simulink model "halfcarmodel"  (R2020b)
settings: Solver=VariableStepAuto  StartTime=0.0  StopTime=10.0  RelTol=1e-3
values from neighbouring files (symbols this model uses):
  a = 1.5    [halfcarparameters.mat]
  b = 1    [accel_jerk_ctrl_testbed.m]    (also in halfcarparameters.mat = 1.5)
  K_tf = 201021    [halfcarparameters.mat]
  K_tr = 201021    [halfcarparameters.mat]
  m_s = 879.35    [halfcarparameters.mat]
settings Model: Creator=anishabhangui  LastModifiedBy=anishabhangui

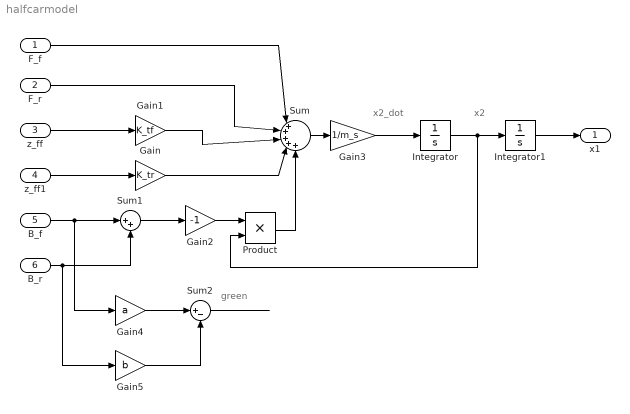
== system halfcarmodel ==
  note: green
  note: x2
  note: x2_dot
  F_f : Inport
  F_r : Inport  Port=2
  z_ff : Inport  Port=3
  z_ff1 : Inport  Port=4
  B_f : Inport  Port=5
  B_r : Inport  Port=6
  Gain : Gain  Gain=K_tr
  Gain1 : Gain  Gain=K_tf
  Gain2 : Gain  Gain=-1
  Gain3 : Gain  Gain=1/m_s
  Gain4 : Gain  Gain=a
  Gain5 : Gain  Gain=b
  Integrator : Integrator
  Integrator1 : Integrator
  Product : Product
  Sum : Sum  Inputs=|+++++
  Sum1 : Sum  Inputs=|++
  Sum2 : Sum  Inputs=|+-
  x1 : Outport
  wires:
  z_ff1/1 -> Gain/1
  z_ff/1 -> Gain1/1
  F_f/1 -> Sum/1
  F_r/1 -> Sum/2
  Gain1/1 -> Sum/3
  Gain/1 -> Sum/4
  Integrator1/1 -> x1/1
  B_f/1 -> Gain4/1, Sum1/1
  B_r/1 -> Gain5/1, Sum1/2
  Sum1/1 -> Gain2/1
  Gain2/1 -> Product/1
  Integrator/1 -> Product/2, Integrator1/1
  Product/1 -> Sum/5
  Sum/1 -> Gain3/1
  Gain3/1 -> Integrator/1
  Gain4/1 -> Sum2/1
  Gain5/1 -> Sum2/2
  Sum2/1 -> ?
